simulink model "Battery_Model"  (R2025a)
settings: Solver=ode4  StartTime=0.0  StopTime=10000  FixedStep=0.01  RelTol=1e-3
settings Model: Creator=asgha  LastModifiedBy=asgha

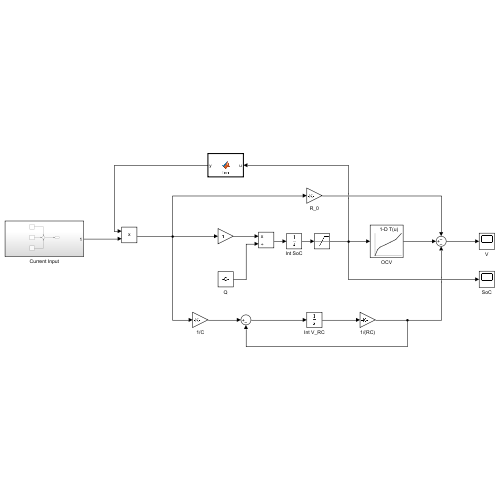
[thumbnail: Simulink's stored preview of the top-level diagram]
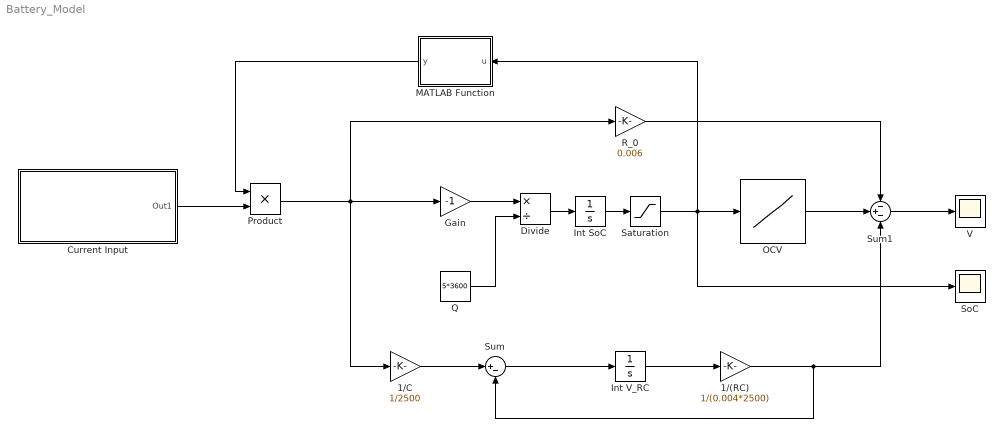
== system Battery_Model ==
  1/(RC) : Gain  Gain=1/(0.004*2500)
  1/C : Gain  Gain=1/2500
  Current Input : Subsystem
  Divide : Product  Inputs=*/
  Gain : Gain  Gain=-1
  Int SoC : Integrator  InitialCondition=1
  Int V_RC : Integrator
  MATLAB Function : MATLAB Function  TreatAsAtomicUnit=on
  OCV : Lookup_n-D  NumberOfTableDimensions=1  BreakpointsForDimension1=[0.0 0.1 0.2 0.4 0.6 0.8 1.0]  Table=[3.30 3.55 3.65 3.75 3.85 3.95 4.20]*4  InternalRulePriority=Speed  RndMeth=Simplest
  Product : Product
  Q : Constant  Value=5*3600
  R_0 : Gain  Gain=0.006
  Saturation : Saturate  UpperLimit=1  LowerLimit=0
  SoC : Scope
      settings: ActiveDisplayYMinimum=-0.068750464897329611  ActiveDisplayYMaximum=1.1187500516552589
  Sum : Sum  Inputs=|+-
  Sum1 : Sum  Inputs=-+-
  V : Scope
      settings: ActiveDisplayYMinimum=13.287860839014217  ActiveDisplayYMaximum=17.170237684553978
  wires:
  Product/1 -> R_0/1, 1/C/1, Gain/1
  Gain/1 -> Divide/1
  Q/1 -> Divide/2
  Divide/1 -> Int SoC/1
  Saturation/1 -> MATLAB Function/1(u), SoC/1, OCV/1
  Sum/1 -> Int V_RC/1
  Int V_RC/1 -> 1/(RC)/1
  1/(RC)/1 -> Sum1/3, Sum/2
  1/C/1 -> Sum/1
  OCV/1 -> Sum1/2
  R_0/1 -> Sum1/1
  Sum1/1 -> V/1
  Int SoC/1 -> Saturation/1
  Current Input/1(Out1) -> Product/2
  MATLAB Function/1(y) -> Product/1

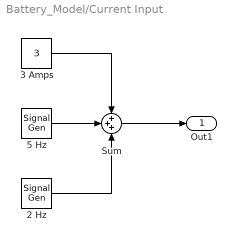
== system Battery_Model/Current Input ==
  2 Hz : SignalGenerator  Amplitude=0.5  Frequency=0.02  Units=rad/sec
  3 Amps : Constant  Value=3
  5 Hz : SignalGenerator  Frequency=0.01  Units=rad/sec
  Sum : Sum  Inputs=+++
  Out1 : Outport
  wires:
  2 Hz/1 -> Sum/3
  5 Hz/1 -> Sum/2
  3 Amps/1 -> Sum/1
  Sum/1 -> Out1/1

== matlab function Battery_Model/MATLAB Function ==
  data: u input; y output
function y = fcn(u)

if u < 0.05
    y = 0;
else
    y = 1;
end
